simulink model "Task3"  (R2025a)
settings: Solver=VariableStepAuto  StartTime=0.0  StopTime=10.0  RelTol=1e-3
libraries: simulink x1
settings Model: Creator=LOQ  LastModifiedBy=LOQ

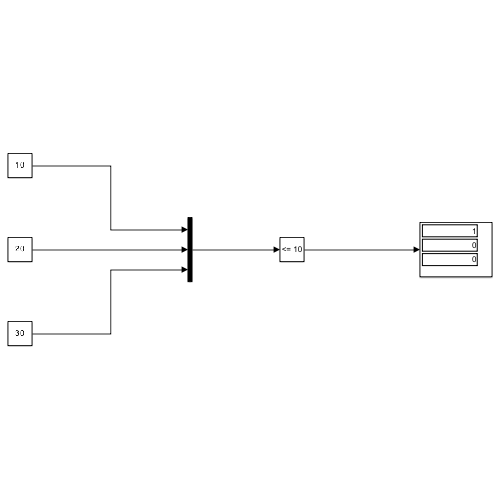
[thumbnail: Simulink's stored preview of the top-level diagram]
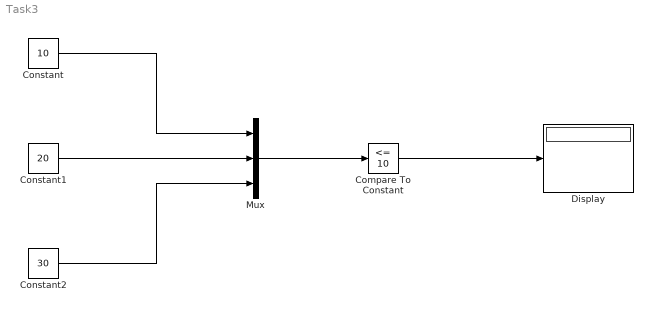
== system Task3 ==
  Compare To Constant : simulink/Logic and Bit Operations/Compare To Constant  relop=<=  const=10  OutDataTypeStr=boolean
  Constant : Constant  Value=10
  Constant1 : Constant  Value=20
  Constant2 : Constant  Value=30
  Display : Display
  Mux : Mux  Inputs=3
  wires:
  Constant1/1 -> Mux/2
  Constant/1 -> Mux/1
  Constant2/1 -> Mux/3
  Mux/1 -> Compare To Constant/1
  Compare To Constant/1 -> Display/1
